simulink library "STATIC_ATT_DET"  (R2021b)
settings: Solver=VariableStepAuto  StartTime=0.0  StopTime=10.0  RelTol=1e-3
undefined symbols (not defined in the file or in its folder): a_vec
libraries: matrix_library x4, vrlib x3, my_math_ops x2
settings Model: Creator=Davide  LastModifiedBy=Davide

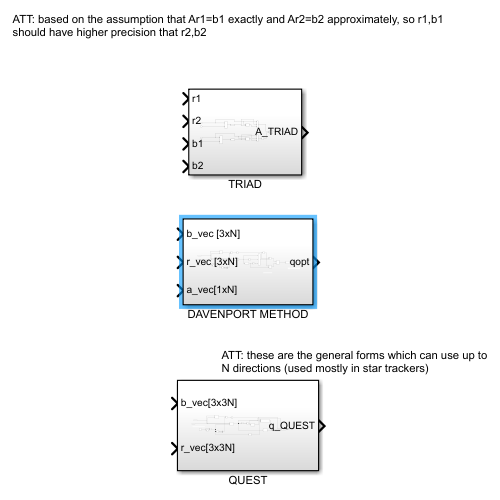
[thumbnail: Simulink's stored preview of the top-level diagram]
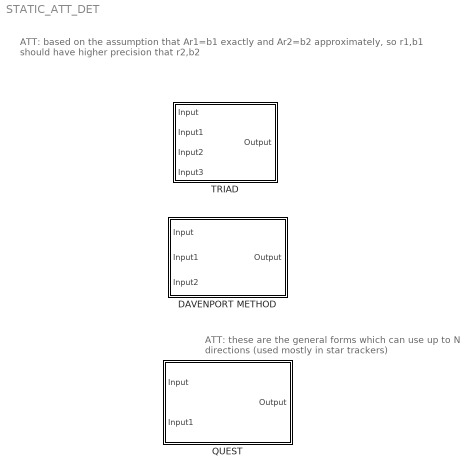
== system STATIC_ATT_DET ==
  note: ATT: these are the general forms which can use up to
      | N directions (used mostly in star trackers)
  note: ATT: based on the assumption that Ar1=b1 exactly and Ar2=b2 approximately, so r1,b1
      | should have higher precision that r2,b2
  DAVENPORT METHOD : Subsystem
  QUEST : Subsystem
  TRIAD : Subsystem

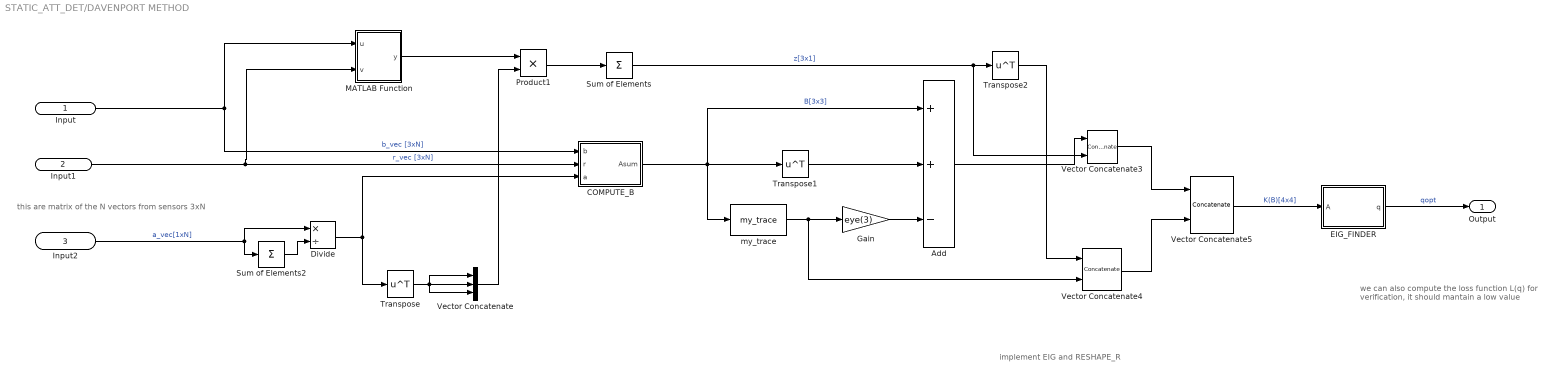
== system STATIC_ATT_DET/DAVENPORT METHOD ==
  note: implement EIG and RESHAPE_R
  note: we can also compute the loss function L(q) for
      | verification, it should mantain a low value
  note: this are matrix of the N vectors from sensors 3xN
  Input : Inport
  Input1 : Inport  Port=2
  Input2 : Inport  Port=3
  Add : Sum  Inputs=++-
  COMPUTE_B : MATLAB Function  TreatAsAtomicUnit=on
  Divide : Product  Inputs=*/
  EIG_FINDER : MATLAB Function  TreatAsAtomicUnit=on
  Gain : Gain  Gain=eye(3)
  MATLAB Function : MATLAB Function  TreatAsAtomicUnit=on
  Product1 : Product
  Sum of Elements : Sum  Inputs=+  CollapseMode=Specified dimension  CollapseDim=2
  Sum of Elements2 : Sum  Inputs=+
  Transpose : Math  Operator=transpose  SaturateOnIntegerOverflow=on
  Transpose1 : Math  Operator=transpose  SaturateOnIntegerOverflow=on
  Transpose2 : Math  Operator=transpose  SaturateOnIntegerOverflow=on
  Vector Concatenate : Concatenate  NumInputs=3  Mode=Multidimensional array
  Vector Concatenate3 : Concatenate  Mode=Multidimensional array  ConcatenateDimension=2
  Vector Concatenate4 : Concatenate  Mode=Multidimensional array  ConcatenateDimension=2
  Vector Concatenate5 : Concatenate  Mode=Multidimensional array
  my_trace : my_math_ops/my_trace  SystemSampleTime=-1  VariantActivationTime=update diagram  Latency=0  AutoFrameSizeCalculation=off
      settings: SourceProductName=My Mathematics Operations
  Output : Outport
  wires:
  EIG_FINDER/1(q) -> Output/1  "qopt"
  COMPUTE_B/1(Asum) -> Add/1, Transpose1/1, my_trace/1  "B[3x3]"
  Sum of Elements/1 -> Vector Concatenate3/2, Transpose2/1  "z[3x1]"
  Input/1 -> COMPUTE_B/1(b), MATLAB Function/1(u)  "b_vec [3xN]"
  Transpose/1 -> Vector Concatenate/1, Vector Concatenate/3, Vector Concatenate/2
  Input1/1 -> MATLAB Function/2(v), COMPUTE_B/2(r)  "r_vec [3xN]"
  Vector Concatenate4/1 -> Vector Concatenate5/2
  Add/1 -> Vector Concatenate3/1
  Transpose2/1 -> Vector Concatenate4/1
  Vector Concatenate3/1 -> Vector Concatenate5/1
  my_trace/1 -> Vector Concatenate4/2, Gain/1
  Transpose1/1 -> Add/2
  Product1/1 -> Sum of Elements/1
  Gain/1 -> Add/3
  Vector Concatenate5/1 -> EIG_FINDER/1(A)  "K(B)[4x4]"
  Vector Concatenate/1 -> Product1/2
  MATLAB Function/1(y) -> Product1/1
  Divide/1 -> COMPUTE_B/3(a), Transpose/1
  Sum of Elements2/1 -> Divide/2
  Input2/1 -> Divide/1, Sum of Elements2/1  "a_vec[1xN]"

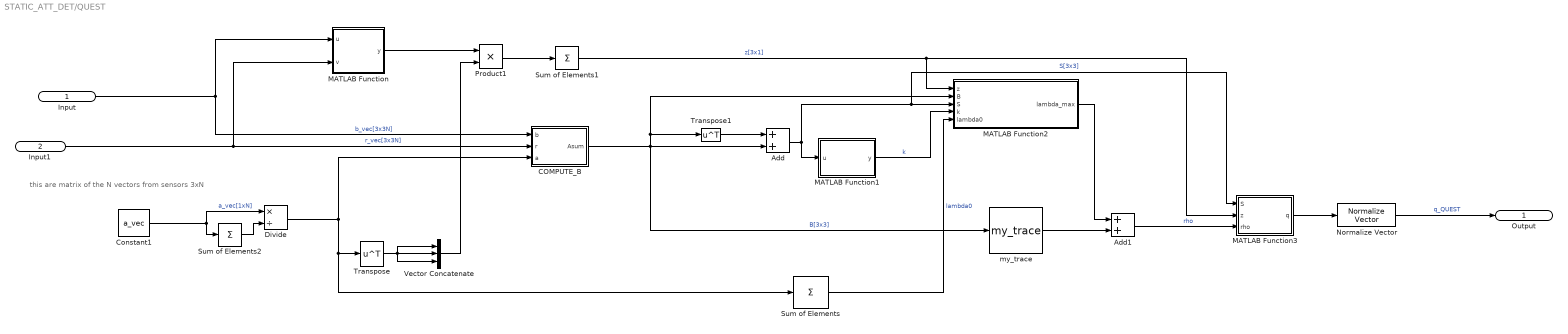
== system STATIC_ATT_DET/QUEST ==
  note: this are matrix of the N vectors from sensors 3xN
  Input : Inport
  Input1 : Inport  Port=2
  Add : Sum
  Add1 : Sum
  COMPUTE_B : MATLAB Function  TreatAsAtomicUnit=on
  Constant1 : Constant  Value=a_vec
  Divide : Product  Inputs=*/
  MATLAB Function : MATLAB Function  TreatAsAtomicUnit=on
  MATLAB Function1 : MATLAB Function  TreatAsAtomicUnit=on
  MATLAB Function2 : MATLAB Function  TreatAsAtomicUnit=on
  MATLAB Function3 : MATLAB Function  TreatAsAtomicUnit=on
  Normalize Vector : vrlib/Utilities/Normalize Vector  maxzero=0
  Product1 : Product
  Sum of Elements : Sum  Inputs=+  CollapseMode=Specified dimension
  Sum of Elements1 : Sum  Inputs=+  CollapseMode=Specified dimension  CollapseDim=2
  Sum of Elements2 : Sum  Inputs=+
  Transpose : Math  Operator=transpose  SaturateOnIntegerOverflow=on
  Transpose1 : Math  Operator=transpose  SaturateOnIntegerOverflow=on
  Vector Concatenate : Concatenate  NumInputs=3  Mode=Multidimensional array
  my_trace : my_math_ops/my_trace  SystemSampleTime=-1  VariantActivationTime=update diagram  Latency=0  AutoFrameSizeCalculation=off
      settings: SourceProductName=My Mathematics Operations
  Output : Outport
  wires:
  Input1/1 -> MATLAB Function/2(v), COMPUTE_B/2(r)  "r_vec[3x3N]"
  Add1/1 -> MATLAB Function3/3(rho)  "rho"
  Transpose/1 -> Vector Concatenate/1, Vector Concatenate/3, Vector Concatenate/2
  Input/1 -> COMPUTE_B/1(b), MATLAB Function/1(u)  "b_vec[3x3N]"
  Product1/1 -> Sum of Elements1/1
  Add/1 -> MATLAB Function3/1(S), MATLAB Function2/3(S), MATLAB Function1/1(u)  "S[3x3]"
  MATLAB Function/1(y) -> Product1/1
  Constant1/1 -> Divide/1, Sum of Elements2/1  "a_vec[1xN]"
  MATLAB Function1/1(y) -> MATLAB Function2/4(k)  "k"
  COMPUTE_B/1(Asum) -> my_trace/1, MATLAB Function2/2(B), Transpose1/1, Add/2  "B[3x3]"
  Vector Concatenate/1 -> Product1/2
  Transpose1/1 -> Add/1
  MATLAB Function3/1(q) -> Normalize Vector/1
  Sum of Elements1/1 -> MATLAB Function3/2(z), MATLAB Function2/1(z)  "z[3x1]"
  MATLAB Function2/1(lambda_max) -> Add1/1
  Sum of Elements/1 -> MATLAB Function2/5(lambda0)  "lambda0"
  my_trace/1 -> Add1/2
  Normalize Vector/1 -> Output/1  "q_QUEST"
  Divide/1 -> COMPUTE_B/3(a), Sum of Elements/1, Transpose/1
  Sum of Elements2/1 -> Divide/2

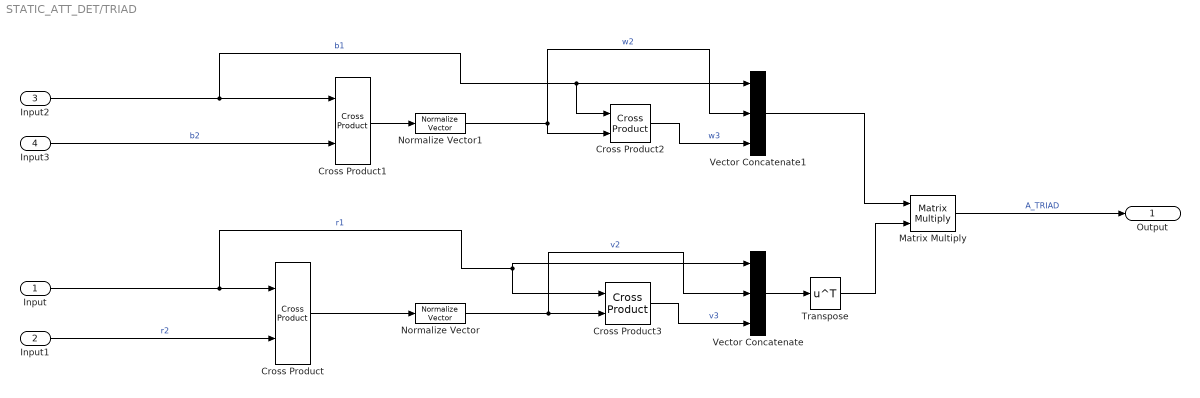
== system STATIC_ATT_DET/TRIAD ==
  Input : Inport
  Input1 : Inport  Port=2
  Input2 : Inport  Port=3
  Input3 : Inport  Port=4
  Cross Product{,1..3} (4 alike) : matrix_library/Cross Product
      settings: SourceProductBaseCode=SL
  Matrix Multiply : Product  Multiplication=Matrix(*)
  Normalize Vector : vrlib/Utilities/Normalize Vector  maxzero=0
  Normalize Vector1 : vrlib/Utilities/Normalize Vector  maxzero=0
  Transpose : Math  Operator=transpose  SaturateOnIntegerOverflow=on
  Vector Concatenate : Concatenate  NumInputs=3  Mode=Multidimensional array  ConcatenateDimension=2
  Vector Concatenate1 : Concatenate  NumInputs=3  Mode=Multidimensional array  ConcatenateDimension=2
  Output : Outport
  wires:
  Matrix Multiply/1 -> Output/1  "A_TRIAD"
  Input/1 -> Cross Product3/1, Vector Concatenate/1, Cross Product/1  "r1"
  Normalize Vector1/1 -> Vector Concatenate1/2, Cross Product2/2  "w2"
  Input1/1 -> Cross Product/2  "r2"
  Cross Product/1 -> Normalize Vector/1
  Input2/1 -> Cross Product2/1, Vector Concatenate1/1, Cross Product1/1  "b1"
  Normalize Vector/1 -> Cross Product3/2, Vector Concatenate/2  "v2"
  Input3/1 -> Cross Product1/2  "b2"
  Cross Product1/1 -> Normalize Vector1/1
  Cross Product3/1 -> Vector Concatenate/3  "v3"
  Cross Product2/1 -> Vector Concatenate1/3  "w3"
  Vector Concatenate/1 -> Transpose/1
  Vector Concatenate1/1 -> Matrix Multiply/1
  Transpose/1 -> Matrix Multiply/2

== matlab function STATIC_ATT_DET/QUEST/COMPUTE_B ==
  data: b input; Asum output; r input; a input
function Asum = fcn(b,r,a)
N = length(a);
Asum = zeros(3);
for i = 1:N
    Asum = Asum + a(i) * b(:,i)*r(:,i)';
end

== matlab function STATIC_ATT_DET/DAVENPORT METHOD/COMPUTE_B ==
  data: b input; Asum output; r input; a input
function Asum = fcn(b,r,a)
N = length(a);
Asum = zeros(3);
for i = 1:N
    Asum = Asum + a(i) * b(:,i)*r(:,i)';
end

== matlab function STATIC_ATT_DET/DAVENPORT METHOD/MATLAB Function ==
  data: u input; y output; v input
function y = fcn(u,v)

y = cross(u,v);

== matlab function STATIC_ATT_DET/DAVENPORT METHOD/EIG_FINDER ==
  data: A input; q output
function q = fcn(A)
[V,D] = eig(A);
[d,ind] = sort(diag(D),'ComparisonMethod', 'real');
V = V(:,ind);
q = real(V(:,4)/norm(V(:,4)));

== matlab function STATIC_ATT_DET/QUEST/MATLAB Function ==
  data: u input; y output; v input
function y = crossN(u,v)

y = cross(u,v);

== matlab function STATIC_ATT_DET/QUEST/MATLAB Function1 ==
  data: u input; y output
function y = fcn(u)

y = trace(det(u)*inv(u));

== matlab function STATIC_ATT_DET/QUEST/MATLAB Function2 ==
  data: z input; B input; lambda_max output; S input; k input; lambda0 input
function lambda_max = fcn(z,B,S,k,lambda0)

lambda_max = fzero(@(l) ((l^2 - trace(B)^2 + k)*(l^2 - trace(B)^2 - norm(z)^2)) - (l-trace(B))*(z'*S*z + det(S)) - z'*S^2*z,lambda0);

== matlab function STATIC_ATT_DET/QUEST/MATLAB Function3 ==
  data: S input; q output; z input; rho input
function q = fcn(S,z,rho)
A = rho*eye(3)-S;
q = [det(A)*A\z; det(A)];
